simulink model "separator_l2"  (R2017b)
settings: Solver=VariableStepAuto  StartTime=0.0  StopTime=100.0  RelTol=1e-3
libraries: simulink x1
settings Model: Creator=Bailey Brookes  LastModifiedBy=Bailey Brookes

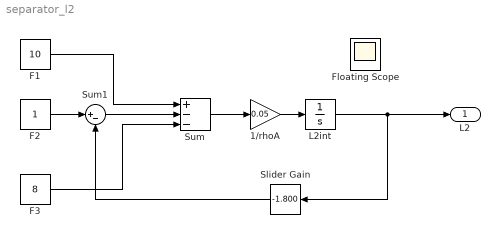
== system separator_l2 ==
  1/rhoA : Gain  Gain=0.05
  F1 : Constant  Value=10
  F2 : Constant
  F3 : Constant  Value=8
  Floating Scope : Scope
      settings: Floating=on
  L2int : Integrator
  Slider Gain : simulink/Math Operations/Slider Gain  gain=-1.800  low=-6  high=0
  Sum : Sum  Inputs=+--
  Sum1 : Sum  Inputs=|+-
  L2 : Outport
  wires:
  1/rhoA/1 -> L2int/1
  F3/1 -> Sum/3
  Sum/1 -> 1/rhoA/1
  F1/1 -> Sum/1
  Slider Gain/1 -> Sum1/2
  Sum1/1 -> Sum/2
  L2int/1 -> Slider Gain/1, L2/1
  F2/1 -> Sum1/1
